simulink model "explicitCompFilter_uORB"  (R2024b)
settings: Solver=FixedStepAuto  StartTime=0.0  StopTime=35  FixedStep=0.005  RelTol=1e-3  EnableMultiTasking=on
PreLoadFcn:
  | %b_prev = Simulink.Signal;
  | %q_prev = Simulink.Signal;
  | 
  | %b_prev.InitialValue = '[0; 0; 0]';
  | %q_prev.InitialValue = '[0; 0; 0; 0]';
InitFcn:
  | %g_or = [0;0;-9.81];
  | %m_or = [27.5550; 2.4169; 16.0849];
  | gyroBias = [1; 1; 0.5];
  | 
  | %IF USING BUILT-IN UAV ANIMATION, uncomment below
  | 
  | %CLEAR UAV ANIMATIONS
  | %figHandles = findall(groot, 'Type', 'figure');
  | 
  | %for i=1:size(figHandles)
  | %    figObj = figHandles(i);
  | %    figName = figObj.Name;
  | %   if contains(figName, 'UAV Animation');
  | %        delete(figObj);
  | %    end
  | %end
undefined symbols (not defined in the file): g
libraries: robotcorelib x3, simulink_extras x3, px4Sensorslib x2, simulink x1, matrix_library x1, vrlib x1, px4uORBlib x1
(part 3 of 3)

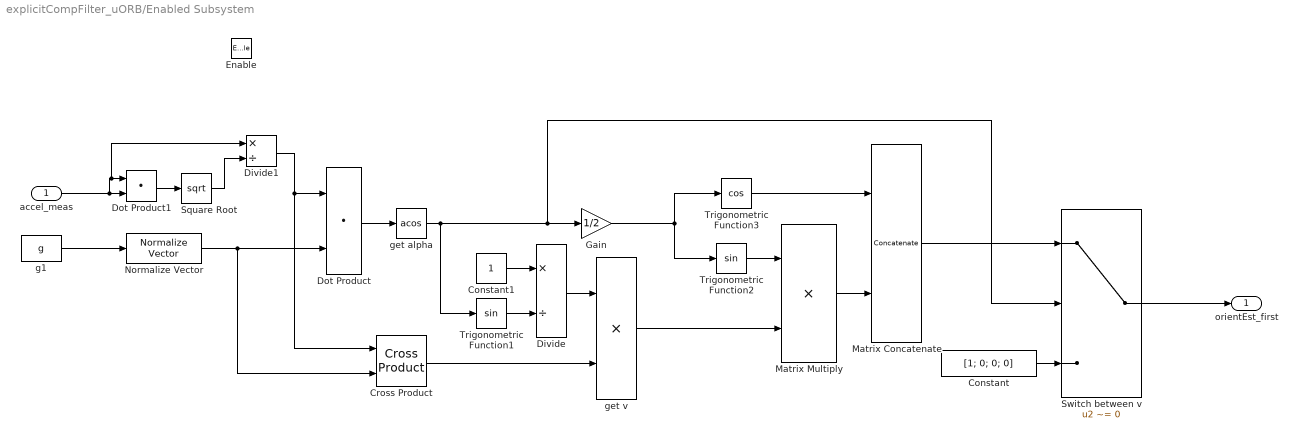
== system explicitCompFilter_uORB/Enabled Subsystem ==
  accel_meas : Inport
  Enable : EnablePort
  Constant : Constant  Value=[1; 0; 0; 0]  VectorParams1D=off
  Constant1 : Constant
  Cross Product : matrix_library/Cross Product
  Divide : Product  Inputs=*/
  Divide1 : Product  Inputs=*/
  Dot Product : DotProduct  OutDataTypeStr=Inherit: Inherit via internal rule
  Dot Product1 : DotProduct  OutDataTypeStr=Inherit: Inherit via internal rule
  Gain : Gain  Gain=1/2
  Matrix Concatenate : Concatenate  Mode=Multidimensional array
  Matrix Multiply : Product
  Normalize Vector : vrlib/Utilities/Normalize Vector  maxzero=0
  Square Root : Sqrt
  Switch between v : Switch  Criteria=u2 ~= 0  SaturateOnIntegerOverflow=off  InputSameDT=off
  Trigonometric Function1 : Trigonometry
  Trigonometric Function2 : Trigonometry  OutputSignalType=real
  Trigonometric Function3 : Trigonometry  Operator=cos  OutputSignalType=real
  g1 : Constant  Value=g  OutDataTypeStr=Inherit: Inherit via back propagation
  get alpha : Trigonometry  Operator=acos
  get v : Product
  orientEst_first : Outport
  wires:
  accel_meas/1 -> Dot Product1/2, Divide1/1, Dot Product1/1
  g1/1 -> Normalize Vector/1
  Square Root/1 -> Divide1/2
  Normalize Vector/1 -> Cross Product/2, Dot Product/2
  Dot Product/1 -> get alpha/1
  Constant/1 -> Switch between v/3
  Constant1/1 -> Divide/1
  Divide/1 -> get v/1
  Trigonometric Function1/1 -> Divide/2
  Cross Product/1 -> get v/2
  get alpha/1 -> Switch between v/2, Gain/1, Trigonometric Function1/1
  Gain/1 -> Trigonometric Function2/1, Trigonometric Function3/1
  Trigonometric Function2/1 -> Matrix Multiply/1
  get v/1 -> Matrix Multiply/2
  Matrix Multiply/1 -> Matrix Concatenate/2
  Trigonometric Function3/1 -> Matrix Concatenate/1
  Matrix Concatenate/1 -> Switch between v/1
  Switch between v/1 -> orientEst_first/1
  Dot Product1/1 -> Square Root/1
  Divide1/1 -> Dot Product/1, Cross Product/1

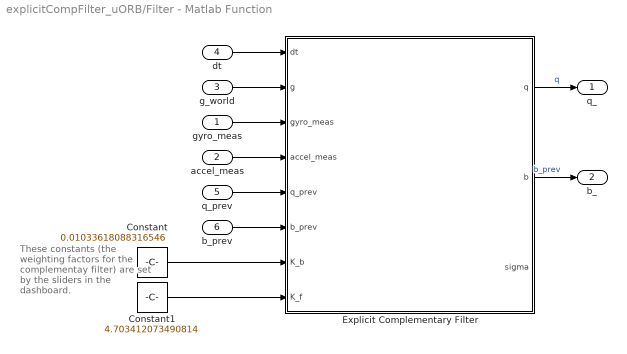
== system explicitCompFilter_uORB/Filter - Matlab Function ==
  note: These constants (the weighting factors for the complementay filter) are set by the sliders in the dashboard.
  gyro_meas : Inport
  accel_meas : Inport  Port=2
  g_world : Inport  Port=3
  dt : Inport  Port=4
  q_prev : Inport  Port=5
  b_prev : Inport  Port=6
  Constant : Constant  Value=0.01033618088316546
  Constant1 : Constant  Value=4.703412073490814
  Explicit Complementary Filter : MATLAB Function  TreatAsAtomicUnit=on
  q_ : Outport
  b_ : Outport  Port=2
  wires:
  g_world/1 -> Explicit Complementary Filter/2(g)
  Explicit Complementary Filter/1(q) -> q_/1  "q"
  gyro_meas/1 -> Explicit Complementary Filter/3(gyro_meas)
  Explicit Complementary Filter/2(b) -> b_/1  "b_prev"
  dt/1 -> Explicit Complementary Filter/1(dt)
  accel_meas/1 -> Explicit Complementary Filter/4(accel_meas)
  Constant1/1 -> Explicit Complementary Filter/8(K_f)
  Constant/1 -> Explicit Complementary Filter/7(K_b)
  q_prev/1 -> Explicit Complementary Filter/5(q_prev)
  b_prev/1 -> Explicit Complementary Filter/6(b_prev)

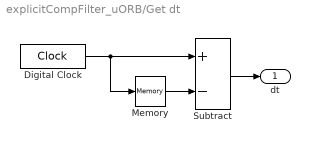
== system explicitCompFilter_uORB/Get dt ==
  Digital Clock : DigitalClock  SampleTime=-1
  Memory : Memory
  Subtract : Sum  Inputs=+-  OutDataTypeStr=Inherit: Inherit via back propagation  InputSameDT=on
  dt : Outport
  wires:
  Digital Clock/1 -> Subtract/1, Memory/1
  Memory/1 -> Subtract/2
  Subtract/1 -> dt/1

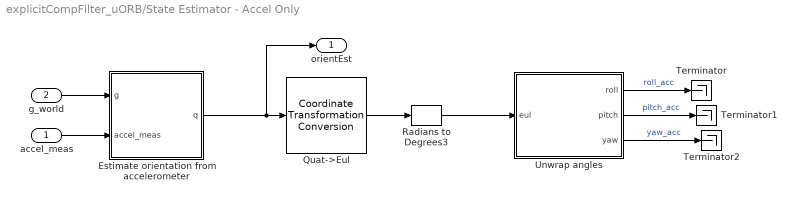
== system explicitCompFilter_uORB/State Estimator - Accel Only ==
  accel_meas : Inport
  g_world : Inport  Port=2
  Estimate orientation from accelerometer : MATLAB Function  TreatAsAtomicUnit=on
  Quat->Eul : robotcorelib/Coordinate Transformation Conversion  InputRepresentation=Quaternion  InputEulerSequence=ZYX  ShowTrVecInputPort=on  OutputRepresentation=Euler Angles  OutputEulerSequence=XYZ  ShowTrVecOutputPort=on  SimulateUsing=Interpreted execution
  Radians to Degrees3 : simulink_extras/Transformations/Radians to Degrees
  Terminator : Terminator
  Terminator1 : Terminator
  Terminator2 : Terminator
  Unwrap angles : MATLAB Function  TreatAsAtomicUnit=on
  orientEst : Outport
  wires:
  Radians to Degrees3/1 -> Unwrap angles/1(eul)
  accel_meas/1 -> Estimate orientation from accelerometer/2(accel_meas)
  Estimate orientation from accelerometer/1(q) -> orientEst/1, Quat->Eul/1
  g_world/1 -> Estimate orientation from accelerometer/1(g)
  Unwrap angles/1(roll) -> Terminator/1  "roll_acc"
  Quat->Eul/1 -> Radians to Degrees3/1
  Unwrap angles/3(yaw) -> Terminator2/1  "yaw_acc"
  Unwrap angles/2(pitch) -> Terminator1/1  "pitch_acc"

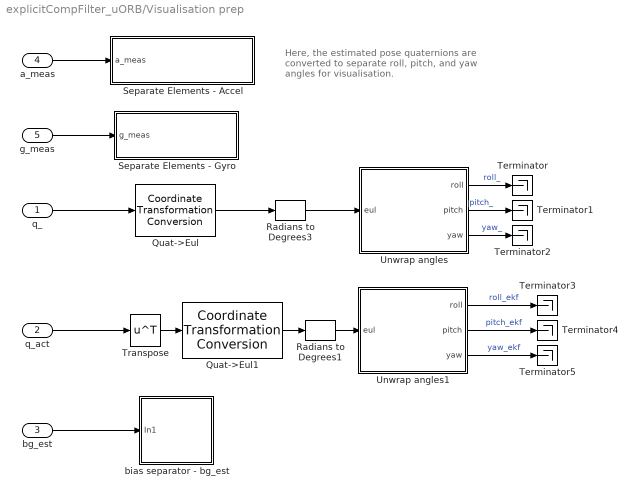
== system explicitCompFilter_uORB/Visualisation prep ==
  note: Here, the estimated pose quaternions are converted to separate roll, pitch, and yaw angles for visualisation.
  q_ : Inport
  q_act : Inport  Port=2
  bg_est : Inport  Port=3
  a_meas : Inport  Port=4
  g_meas : Inport  Port=5
  Quat->Eul : robotcorelib/Coordinate Transformation Conversion  InputRepresentation=Quaternion  InputEulerSequence=ZYX  ShowTrVecInputPort=on  OutputRepresentation=Euler Angles  OutputEulerSequence=XYZ  ShowTrVecOutputPort=on  SimulateUsing=Interpreted execution
  Quat->Eul1 : robotcorelib/Coordinate Transformation Conversion  InputRepresentation=Quaternion  InputEulerSequence=ZYX  ShowTrVecInputPort=on  OutputRepresentation=Euler Angles  OutputEulerSequence=XYZ  ShowTrVecOutputPort=on  SimulateUsing=Interpreted execution
  Radians to Degrees1 : simulink_extras/Transformations/Radians to Degrees
  Radians to Degrees3 : simulink_extras/Transformations/Radians to Degrees
  Separate Elements - Accel : Subsystem
  Separate Elements - Gyro : Subsystem
  Terminator{,1..5} (6 alike) : Terminator
  Transpose : Math  Operator=transpose
  Unwrap angles : MATLAB Function  TreatAsAtomicUnit=on
  Unwrap angles1 : MATLAB Function  TreatAsAtomicUnit=on
  bias separator - bg_est : Subsystem
  wires:
  Transpose/1 -> Quat->Eul1/1
  a_meas/1 -> Separate Elements - Accel/1(a_meas)
  g_meas/1 -> Separate Elements - Gyro/1(g_meas)
  bg_est/1 -> bias separator - bg_est/1(In1)
  q_/1 -> Quat->Eul/1
  q_act/1 -> Transpose/1
  Quat->Eul/1 -> Radians to Degrees3/1
  Quat->Eul1/1 -> Radians to Degrees1/1
  Radians to Degrees3/1 -> Unwrap angles/1(eul)
  Radians to Degrees1/1 -> Unwrap angles1/1(eul)
  Unwrap angles/1(roll) -> Terminator/1  "roll_"
  Unwrap angles/2(pitch) -> Terminator1/1  "pitch_"
  Unwrap angles/3(yaw) -> Terminator2/1  "yaw_"
  Unwrap angles1/3(yaw) -> Terminator5/1  "yaw_ekf"
  Unwrap angles1/2(pitch) -> Terminator4/1  "pitch_ekf"
  Unwrap angles1/1(roll) -> Terminator3/1  "roll_ekf"

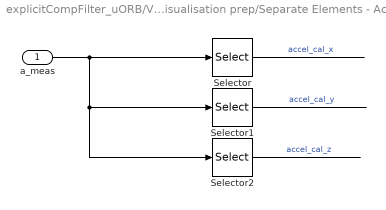
== system explicitCompFilter_uORB/Visualisation prep/Separate Elements - Accel ==
  a_meas : Inport
  Selector : Selector  InputPortWidth=3  IndexOptions=Index vector (dialog)  Indices=[1]  OutputSizes=1
  Selector1 : Selector  InputPortWidth=3  IndexOptions=Index vector (dialog)  Indices=[2]  OutputSizes=1
  Selector2 : Selector  InputPortWidth=3  IndexOptions=Index vector (dialog)  Indices=[3]  OutputSizes=1
  wires:
  a_meas/1 -> Selector/1, Selector1/1, Selector2/1
  Selector1/1 -> ?  "accel_cal_y"
  Selector2/1 -> ?  "accel_cal_z"
  Selector/1 -> ?  "accel_cal_x"

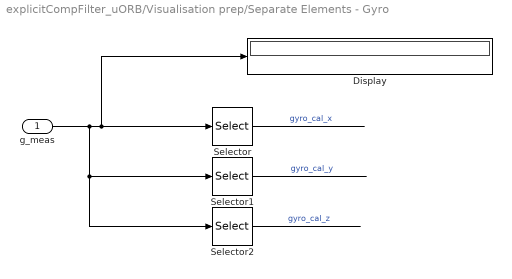
== system explicitCompFilter_uORB/Visualisation prep/Separate Elements - Gyro ==
  g_meas : Inport
  Display : Display
  Selector : Selector  InputPortWidth=3  IndexOptions=Index vector (dialog)  Indices=[1]  OutputSizes=1
  Selector1 : Selector  InputPortWidth=3  IndexOptions=Index vector (dialog)  Indices=[2]  OutputSizes=1
  Selector2 : Selector  InputPortWidth=3  IndexOptions=Index vector (dialog)  Indices=[3]  OutputSizes=1
  wires:
  Selector/1 -> ?  "gyro_cal_x"
  Selector2/1 -> ?  "gyro_cal_z"
  Selector1/1 -> ?  "gyro_cal_y"
  g_meas/1 -> Selector2/1, Selector1/1, Display/1, Selector/1

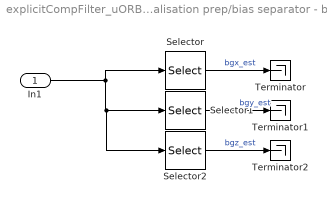
== system explicitCompFilter_uORB/Visualisation prep/bias separator - bg_est ==
  In1 : Inport
  Selector : Selector  InputPortWidth=3  IndexOptions=Index vector (dialog)  Indices=1  OutputSizes=1
  Selector1 : Selector  InputPortWidth=3  IndexOptions=Index vector (dialog)  Indices=2  OutputSizes=1
  Selector2 : Selector  InputPortWidth=3  IndexOptions=Index vector (dialog)  Indices=1  OutputSizes=1
  Terminator : Terminator
  Terminator1 : Terminator
  Terminator2 : Terminator
  wires:
  Selector/1 -> Terminator/1  "bgx_est"
  In1/1 -> Selector/1, Selector2/1, Selector1/1
  Selector1/1 -> Terminator1/1  "bgy_est"
  Selector2/1 -> Terminator2/1  "bgz_est"

== matlab function explicitCompFilter_uORB/State Estimator - Accel Only/Unwrap angles ==
  data: eul input; roll output; pitch output; yaw output
function [roll, pitch, yaw] = fcn(eul)

phi = eul(1);
theta = eul(2);
psi = eul(3);

% x-
% if phi < 0
%     roll = phi+360;
% else
%     roll = phi;
% end
if phi>180
    roll = phi - 360;
elseif phi<-180
    roll = phi + 360;
else
    roll = phi;
end

% y-
if theta>180
    pitch = theta - 360;
elseif theta<-180
    pitch = theta + 360;
else
    pitch = theta;
end

% z- 
% if psi < 0
%     yaw = psi+360;
% else
%     yaw = psi;
% end
if psi>180
    yaw = psi - 360;
elseif psi<-180
    yaw = psi + 360;
else
    yaw = psi;
end

== matlab function explicitCompFilter_uORB/Filter - Matlab Function/Explicit Complementary Filter ==
  data: dt input; g input; gyro_meas input; q output size=[4,1]; accel_meas input; q_prev input; b_prev input; b output; K_b input; K_f input; sigma output
function [q, b, sigma] = fcn(dt, g, gyro_meas, accel_meas, q_prev, b_prev, K_b, K_f)

%% PRELIMINARIES
q = zeros(4,1);
accel_meas_dbl = double(accel_meas);
gyro_meas_dbl = double(gyro_meas);

%% INITIALISATION
% If running for the first time, initialise with some pose estimate from
% the accelerometer
if q_prev == [0; 0; 0; 0]
    accel_meas_hat = accel_meas_dbl/norm(accel_meas_dbl); % normalise acceleration measurement
    g_hat = g/norm(g);
    alpha = acos(dot(accel_meas_hat, g_hat));
    if alpha == 0
        q_prev = [1; 0; 0; 0];
    else
        v = cross(accel_meas_hat, g_hat);
        v = 1/sin(alpha) * v;
        q_prev = ([cos(alpha/2); v*sin(alpha/2)]);
    end 
end

%% ORIENTATION ERROR

%compare accelerometer measurement to estimated gravity vector direction
accel_meas_hat = accel_meas/norm(accel_meas); % normalise acceleration measurement
R_b2w = quat2rotm(q_prev'); %R_b2w
g_bodyframe = R_b2w'*g; %put g in body frame (based on current orientation estimate)
sigma_a = cross( accel_meas_hat,g_bodyframe ); %accelerometer-predicted orientation error

%total error
sigma = sigma_a;

%% GYRO BIAS ESTIMATE
b = double(b_prev - (K_b * sigma)); %Estimate bias

%% ORIENTATION ESTIMATE

% Estimate incremental orientation change
theta = double((gyro_meas_dbl - b + (K_f * sigma)) * dt);
alpha = norm(theta);
if( alpha == 0)
    v = [0; 0; 0];
else
    v = theta/alpha;
end

dq = [cos(alpha/2); sin(alpha/2)*v]; % incremental quaternion
q = quatmultiply(q_prev', dq')'; % next orientation estimate
q = q/norm(q); % normalise


end

== matlab function explicitCompFilter_uORB/Visualisation prep/Unwrap angles ==
  data: eul input; roll output; pitch output; yaw output
function [roll, pitch, yaw] = fcn(eul)

phi = eul(1);
theta = eul(2);
psi = eul(3);

% x-
% if phi < 0
%     roll = phi+360;
% else
%     roll = phi;
% end
if phi>180
    roll = phi - 360;
elseif phi<-180
    roll = phi + 360;
else
    roll = phi;
end

% y-
if theta>180
    pitch = theta - 360;
elseif theta<-180
    pitch = theta + 360;
else
    pitch = theta;
end

% z- 
% if psi < 0
%     yaw = psi+360;
% else
%     yaw = psi;
% end
if psi>180
    yaw = psi - 360;
elseif psi<-180
    yaw = psi + 360;
else
    yaw = psi;
end

== matlab function explicitCompFilter_uORB/Visualisation prep/Unwrap angles1 ==
  data: eul input; roll output; pitch output; yaw output
function [roll, pitch, yaw] = fcn(eul)

phi = eul(1);
theta = eul(2);
psi = eul(3);

% x-
% if phi < 0
%     roll = phi+360;
% else
%     roll = phi;
% end
if phi>180
    roll = phi - 360;
elseif phi<-180
    roll = phi + 360;
else
    roll = phi;
end

% y-
if theta>180
    pitch = theta - 360;
elseif theta<-180
    pitch = theta + 360;
else
    pitch = theta;
end

% z- 
% if psi < 0
%     yaw = psi+360;
% else
%     yaw = psi;
% end
if psi>180
    yaw = psi - 360;
elseif psi<-180
    yaw = psi + 360;
else
    yaw = psi;
end

== matlab function explicitCompFilter_uORB/State Estimator - Accel Only/Estimate orientation from accelerometer ==
  data: g input; q output; accel_meas input
function q = fcn(g, accel_meas)

    accel_meas_dbl = double(accel_meas); 

    accel_meas_hat = accel_meas_dbl/norm(accel_meas_dbl); % normalise acceleration measurement
    g_hat = g/norm(g);
    alpha = acos(dot(accel_meas_hat, g_hat));
    if alpha == 0
        q = [1; 0; 0; 0];
    else
        v = cross(accel_meas_hat, g_hat);
        v = 1/sin(alpha) * v;
        q = [cos(alpha/2); v*sin(alpha/2)];
    end 

end

% function q_est = fcn(q_prev, g, accel_meas)
% 
% 
% accel_meas_dbl = double(accel_meas); 
% 
% %% INITIALISATION
% % If running for the first time, get a first pose estimate from
% % the accelerometer
% if q_prev == [0; 0; 0; 0]
%     accel_meas_hat = accel_meas_dbl/norm(accel_meas_dbl); % normalise acceleration measurement
%     g_hat = g/norm(g);
%     alpha = acos(dot(accel_meas_hat, g_hat));
%     if alpha == 0
%         q_est = double([1; 0; 0; 0]);
%     else
%         v = cross(accel_meas_hat, g_hat);
%         v = 1/sin(alpha) * v;
%         q_est = [cos(alpha/2); v*sin(alpha/2)];
%     end 
% else
%     q_est = double(q_prev);
% end
